simulink model "Simulink"  (R2023b)
settings: Solver=FixedStepAuto  StartTime=0.0  StopTime=10.0  FixedStep=0.00001  RelTol=1e-120
values from neighbouring files (symbols this model uses):
  Bl = 4.2    [Problematique.m]
  c = 340    [Problematique.m]
  d = 1    [Problematique.m]
  Km = 400    [Problematique.m]
  Le = 0.05e-3    (= 5e-05)    [Problematique.m]
  Mm = 10.5e-3    (= 0.0105)    [Problematique.m]
  Re = 3    [Problematique.m]
  rho = 1    [Problematique.m]
  Rm = 0.48    [Problematique.m]
  Rs = 70    [Problematique.m]
  Sm = 0.0222    [Problematique.m]
settings Model: Creator=Martin Chavire  LastModifiedBy=Martin Chavire

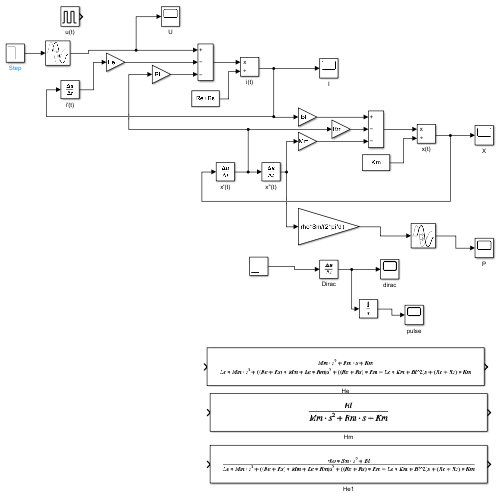
[thumbnail: Simulink's stored preview of the top-level diagram]
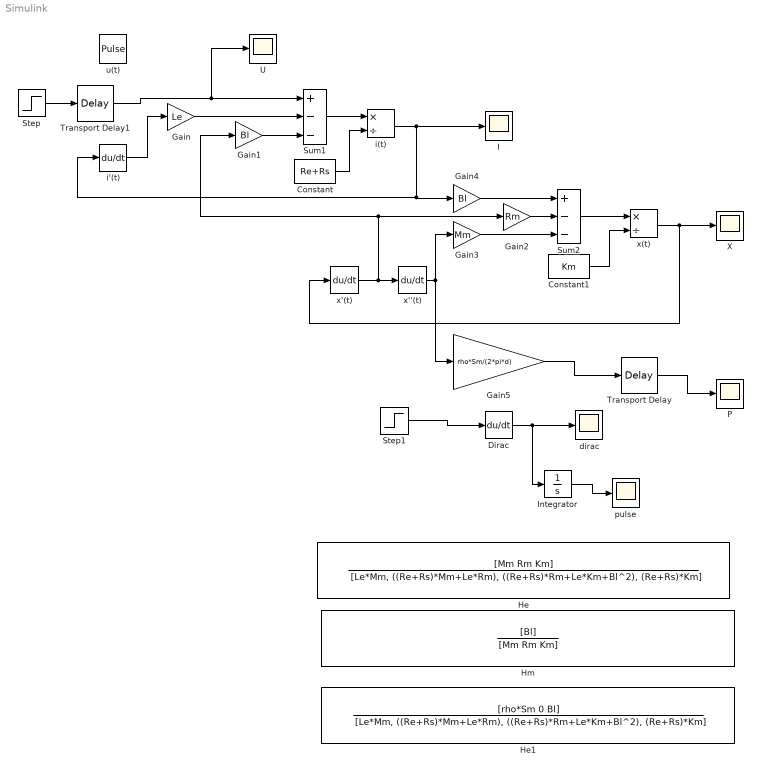
== system Simulink ==
  Constant : Constant  Value=Re+Rs
  Constant1 : Constant  Value=Km
  Dirac : Derivative
  Gain : Gain  Gain=Le
  Gain1 : Gain  Gain=Bl
  Gain2 : Gain  Gain=Rm
  Gain3 : Gain  Gain=Mm
  Gain4 : Gain  Gain=Bl
  Gain5 : Gain  Gain=rho*Sm/(2*pi*d)
  He : TransferFcn  Numerator=[Mm Rm Km]  Denominator=[Le*Mm, ((Re+Rs)*Mm+Le*Rm), ((Re+Rs)*Rm+Le*Km+Bl^2), (Re+Rs)*Km]
  He1 : TransferFcn  Numerator=[rho*Sm 0 Bl]  Denominator=[Le*Mm, ((Re+Rs)*Mm+Le*Rm), ((Re+Rs)*Rm+Le*Km+Bl^2), (Re+Rs)*Km]
  Hm : TransferFcn  Numerator=[Bl]  Denominator=[Mm Rm Km]
  I : Scope
  Integrator : Integrator
  P : Scope
  Step : Step  Time=0.01  Before=3.3  After=0  SampleTime=0
  Step1 : Step  Time=d/c  SampleTime=0
  Sum1 : Sum  Inputs=+--
  Sum2 : Sum  Inputs=+--
  Transport Delay : TransportDelay  DelayTime=d/c
  Transport Delay1 : TransportDelay  DelayTime=5
  U : Scope
  X : Scope
  dirac : Scope
  i'(t) : Derivative
  i(t) : Product  Inputs=*/
  pulse : Scope
  u(t) : DiscretePulseGenerator  PulseType=Time based  Amplitude=3.3  Period=0.01  PulseWidth=50
  x''(t) : Derivative
  x'(t) : Derivative
  x(t) : Product  Inputs=*/
  wires:
  Constant/1 -> i(t)/2
  Gain/1 -> Sum1/2
  Gain1/1 -> Sum1/3
  Sum1/1 -> i(t)/1
  i'(t)/1 -> Gain/1
  i(t)/1 -> i'(t)/1, Gain4/1, I/1
  Gain3/1 -> Sum2/3
  x(t)/1 -> X/1, x'(t)/1
  Sum2/1 -> x(t)/1
  x'(t)/1 -> x''(t)/1, Gain2/1, Gain1/1
  Gain2/1 -> Sum2/2
  Constant1/1 -> x(t)/2
  Gain4/1 -> Sum2/1
  x''(t)/1 -> Gain5/1, Gain3/1
  Step1/1 -> Dirac/1
  Gain5/1 -> Transport Delay/1
  Dirac/1 -> dirac/1, Integrator/1
  Integrator/1 -> pulse/1
  Transport Delay/1 -> P/1
  Step/1 -> Transport Delay1/1
  Transport Delay1/1 -> U/1, Sum1/1
